simulink model "RobotControl1"  (R2015a)
settings: Solver=ode3  StartTime=0.0  StopTime=inf  FixedStep=1/7.5  RelTol=1e-3
undefined symbols (not defined in the file or in its folder): RGB24
libraries: slrtlib x12, xpcvideousblib x3, AAxpcseriallibold x3, xpcobsoletelib x2, rtvideolib x1, xpcutilitieslib x1
settings Model: SimulationMode=external  Creator=farbod  LastModifiedBy=sd0016
settings SolverCC: EnableConcurrentExecution=on
settings DataIOCC: SignalLoggingSaveFormat=ModelDataLogs
settings OptimizationCC: BlockReduction=off  OptimizeBlockIOStorage=off  BufferReuse=off  GlobalBufferReuse=off  ExpressionFolding=off  ExpressionDepthLimit=2147483647  LocalBlockOutputs=off
settings DebuggingCC: UnderspecifiedInitializationDetection=Classic  MergeDetectMultiDrivingBlocksExec=none  FcnCallInpInsideContextMsg=UseLocalSettings  StateNameClashWarn=warning
settings HardwareCC: ProdIntDivRoundTo=Zero  ProdEndianess=LittleEndian  ProdLongLongMode=on  ProdHWDeviceType=Generic->32-bit x86 compatible  TargetBitPerLong=64  TargetBitPerPointer=64  TargetIntDivRoundTo=Zero  TargetEndianess=LittleEndian  TargetWordSize=64  TargetHWDeviceType=Intel->x86-64
settings SFSimCC: SimParseCustomCode=off
settings RTWCC: SystemTargetFile=slrt.tlc  TemplateMakefile=slrt_default_tmf  Description=Simulink Real-Time  RTWVerbose=off  RTWCompilerOptimization=on
settings CodeAppCC: MaxIdLength=95
settings SimulinkRealTimeCC: GeneratePreprocessorConditionals=Disable all

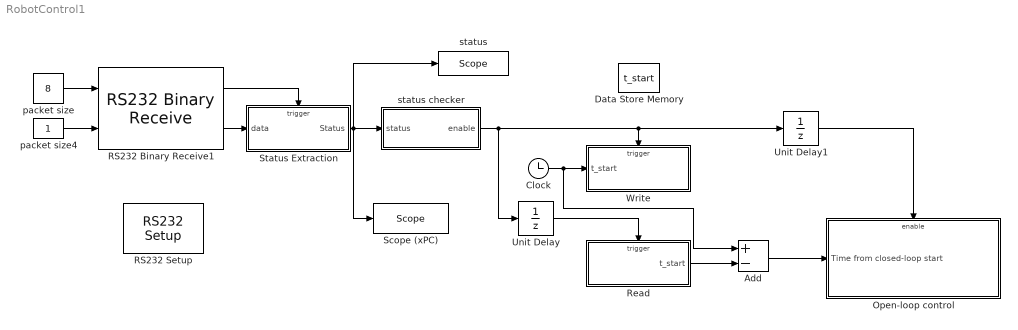
== system RobotControl1 ==
  Add : Sum  Inputs=+-
  Clock : Clock
  Data Store Memory : DataStoreMemory  DataStoreName=t_start  ReadBeforeWriteMsg=warning  WriteAfterWriteMsg=warning  WriteAfterReadMsg=warning
  Open-loop control : Subsystem
  RS232 Binary Receive1 : AAxpcseriallibold/Obsolete/Binary Mode/RS232 Binary Receive  port=COM1  width=8  samptime=-1
  "RS232 Setup " : AAxpcseriallibold/Obsolete/RS232 Setup   port=COM1  baud=115200  dbits=8  sbits=1  parity=None  prot=None  sbuf=2048  rbuf=2048  initstruct=[]  termstruct=[]
  Read : Subsystem  TreatAsAtomicUnit=on
  "Scope (xPC) " : slrtlib/Displays and Logging/Scope   scopeno=20  scopetype=Target  autostart=on  viewmode=Graphical rolling  formatstr='status=%3.3f'  grid=on  ylimits=[0,0]  nosamples=2000  noprepostsamples=0  interleave=1  triggermode=FreeRun  triggersignal=1  trigsignalfromport=off  triggerlevel=0.0  triggerslope=Either  triggerscope=1  triggersample=0  filename=data.dat  mode=Lazy  writesize=512  autorestart=off  dynamicfilemode=off  maxwritefilesize=512*1024^2
  Status Extraction : Subsystem  TreatAsAtomicUnit=on
  Unit Delay : UnitDelay  SampleTime=-1
  Unit Delay1 : UnitDelay  SampleTime=-1
  Write : Subsystem  TreatAsAtomicUnit=on
  packet size : Constant  Value=8
  packet size4 : Constant
  status : slrtlib/Displays and Logging/Scope   scopeno=6  scopetype=File  autostart=on  viewmode=Graphical rolling  formatstr='%15.6f'  grid=on  ylimits=[-10,50]  nosamples=3000  noprepostsamples=0  interleave=1  triggermode=FreeRun  triggersignal=1  trigsignalfromport=off  triggerlevel=0.0  triggerslope=Either  triggerscope=1  triggersample=0  filename=1sttus01.dat  mode=Commit  writesize=512  autorestart=on  dynamicfilemode=off  maxwritefilesize=512*1024^2
  status checker : MATLAB Function  TreatAsAtomicUnit=on
  wires:
  Unit Delay/1 -> Read/Trigger
  Clock/1 -> Write/1(t_start), Add/1
  Read/1(t_start) -> Add/2
  Status Extraction/1(Status) -> status/1, "Scope (xPC) "/1, status checker/1(status)
  status checker/1(enable) -> Write/Trigger, Unit Delay1/1, Unit Delay/1
  Unit Delay1/1 -> Open-loop control/Enable
  Add/1 -> Open-loop control/1(Time from closed-loop start)
  RS232 Binary Receive1/2 -> Status Extraction/1(data)
  RS232 Binary Receive1/1 -> Status Extraction/Trigger
  packet size4/1 -> RS232 Binary Receive1/2
  packet size/1 -> RS232 Binary Receive1/1

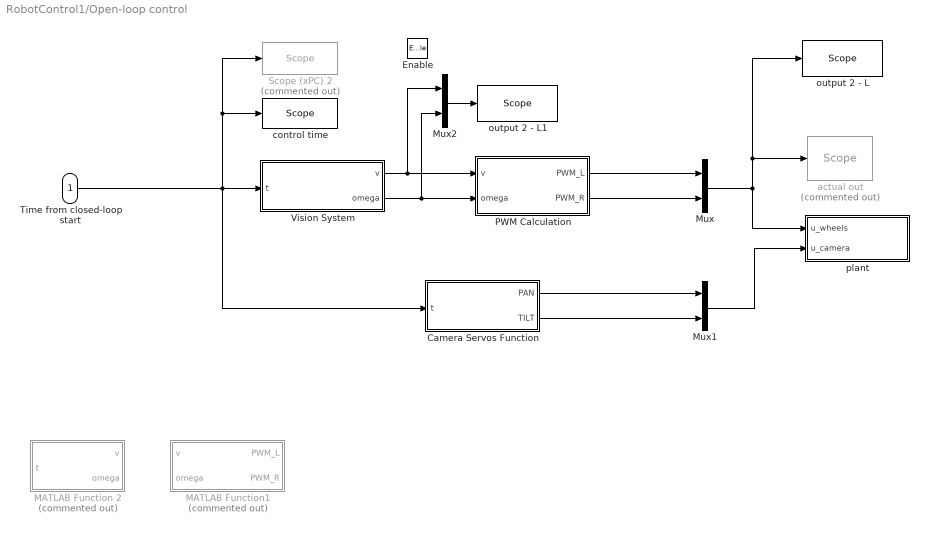
== system RobotControl1/Open-loop control ==
  Time from closed-loop start : Inport
  Enable : EnablePort  PropagateVarSize=During execution
  " MATLAB Function1" : MATLAB Function  Commented=on  TreatAsAtomicUnit=on
  Camera Servos Function : MATLAB Function  TreatAsAtomicUnit=on
  MATLAB Function 2 : MATLAB Function  Commented=on  TreatAsAtomicUnit=on
  Mux : Mux  Inputs=2
  Mux1 : Mux  Inputs=2
  Mux2 : Mux  Inputs=2
  PWM Calculation : MATLAB Function  TreatAsAtomicUnit=on
  Scope (xPC) 2 : slrtlib/Displays and Logging/Scope   Commented=on  scopeno=1  scopetype=File  autostart=on  viewmode=Graphical redraw  formatstr='%15.6f'  grid=on  ylimits=[0,0]  nosamples=3000  noprepostsamples=0  interleave=1  triggermode=FreeRun  triggersignal=1  trigsignalfromport=off  triggerlevel=0.0  triggerslope=Either  triggerscope=1  triggersample=0  filename=1ctime01.dat  mode=Commit  writesize=512  autorestart=off  dynamicfilemode=off  maxwritefilesize=512*1024^2
  Vision System : Subsystem
  actual out : slrtlib/Displays and Logging/Scope   Commented=on  scopeno=7  scopetype=File  autostart=on  viewmode=Graphical rolling  formatstr='%15.6f'  grid=on  ylimits=[-3,150]  nosamples=3000  noprepostsamples=0  interleave=1  triggermode=FreeRun  triggersignal=1  trigsignalfromport=off  triggerlevel=0.0  triggerslope=Either  triggerscope=1  triggersample=0  filename=1pwm01.dat  mode=Commit  writesize=512  autorestart=on  dynamicfilemode=off  maxwritefilesize=512*1024^2
  control time : slrtlib/Displays and Logging/Scope   scopeno=15  scopetype=Target  autostart=on  viewmode=Numerical  formatstr='t=%3.3f'  grid=on  ylimits=[0,0]  nosamples=3  noprepostsamples=0  interleave=1  triggermode=FreeRun  triggersignal=1  trigsignalfromport=off  triggerlevel=0.0  triggerslope=Either  triggerscope=1  triggersample=0  filename=data.dat  mode=Lazy  writesize=512  autorestart=off  dynamicfilemode=off  maxwritefilesize=512*1024^2
  output 2 - L : slrtlib/Displays and Logging/Scope   scopeno=11  scopetype=Target  autostart=on  viewmode=Numerical  formatstr='%15.6f'  grid=on  ylimits=[0,0]  nosamples=3  noprepostsamples=0  interleave=1  triggermode=FreeRun  triggersignal=1  trigsignalfromport=off  triggerlevel=0.0  triggerslope=Either  triggerscope=1  triggersample=0  filename=data.dat  mode=Lazy  writesize=512  autorestart=off  dynamicfilemode=off  maxwritefilesize=512*1024^2
  output 2 - L1 : slrtlib/Displays and Logging/Scope   scopeno=10  scopetype=Target  autostart=on  viewmode=Numerical  formatstr='%15.6f'  grid=on  ylimits=[0,0]  nosamples=3  noprepostsamples=0  interleave=1  triggermode=FreeRun  triggersignal=1  trigsignalfromport=off  triggerlevel=0.0  triggerslope=Either  triggerscope=1  triggersample=0  filename=data.dat  mode=Lazy  writesize=512  autorestart=off  dynamicfilemode=off  maxwritefilesize=512*1024^2
  plant : Subsystem
  wires:
  Mux/1 -> output 2 - L/1, actual out/1, plant/1(u_wheels)
  Camera Servos Function/1(PAN) -> Mux1/1
  Camera Servos Function/2(TILT) -> Mux1/2
  Mux1/1 -> plant/2(u_camera)
  PWM Calculation/1(PWM_L) -> Mux/1
  PWM Calculation/2(PWM_R) -> Mux/2
  Time from closed-loop start/1 -> Vision System/1(t), Scope (xPC) 2/1, control time/1, Camera Servos Function/1(t)
  Vision System/2(omega) -> Mux2/2, PWM Calculation/2(omega)
  Vision System/1(v) -> Mux2/1, PWM Calculation/1(v)
  Mux2/1 -> output 2 - L1/1

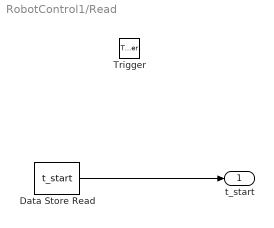
== system RobotControl1/Read ==
  Trigger : TriggerPort
  Data Store Read : DataStoreRead  DataStoreName=t_start
  t_start : Outport
  wires:
  Data Store Read/1 -> t_start/1

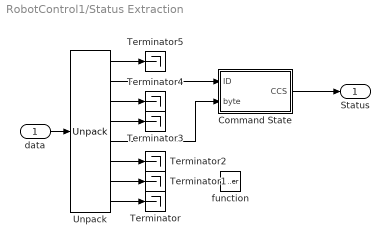
== system RobotControl1/Status Extraction ==
  data : Inport
  function : TriggerPort  TriggerType=function-call  OutputDataType=int8
  Command State : MATLAB Function  TreatAsAtomicUnit=on
  Terminator{,1..5} (6 alike) : Terminator
  Unpack : xpcobsoletelib/Utilities/Unpack   dimensions={1,1,1,1,1,1,1,1}  datatypes={'uint8','uint8','uint8','uint8','uint8','uint8','uint8','uint8'}  byteAlign=1
  Status : Outport
  wires:
  data/1 -> Unpack/1
  Command State/1(CCS) -> Status/1
  Unpack/5 -> Command State/2(byte)
  Unpack/2 -> Command State/1(ID)
  Unpack/8 -> Terminator/1
  Unpack/1 -> Terminator5/1
  Unpack/3 -> Terminator4/1
  Unpack/4 -> Terminator3/1
  Unpack/6 -> Terminator2/1
  Unpack/7 -> Terminator1/1

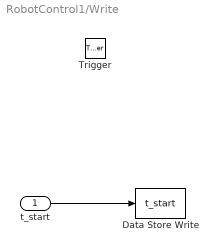
== system RobotControl1/Write ==
  t_start : Inport
  Trigger : TriggerPort
  Data Store Write : DataStoreWrite  DataStoreName=t_start
  wires:
  t_start/1 -> Data Store Write/1

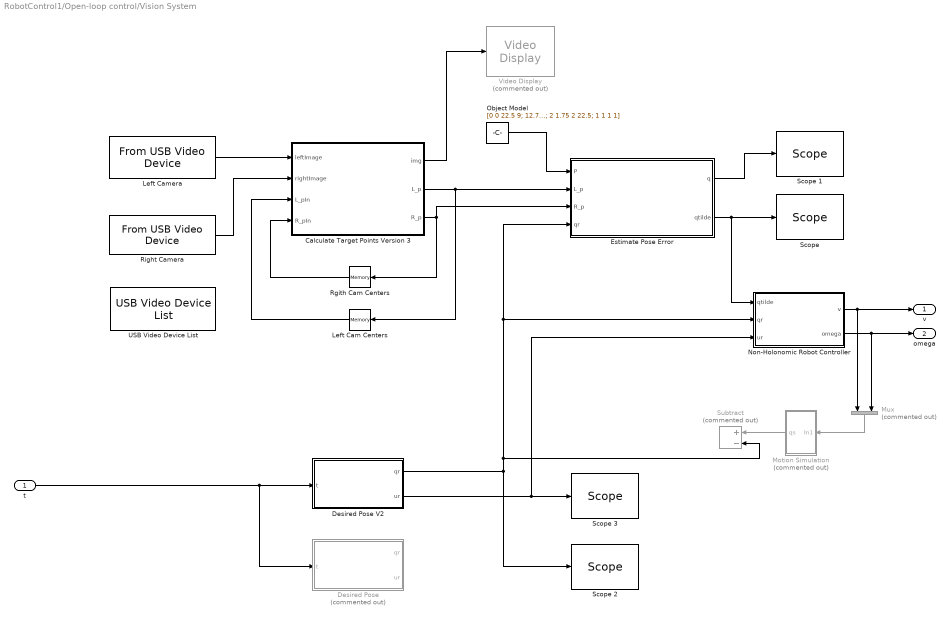
== system RobotControl1/Open-loop control/Vision System ==
  t : Inport
  Calculate Target Points Version 3 : MATLAB Function  TreatAsAtomicUnit=on
  Desired Pose : MATLAB Function  Commented=on  TreatAsAtomicUnit=on
  Desired Pose V2 : MATLAB Function  TreatAsAtomicUnit=on
  Estimate Pose Error : MATLAB Function  TreatAsAtomicUnit=on
  Left Cam Centers : Memory  X0=|  InheritSampleTime=on
      | [648.8644  845.2955  739.9159  733.5896;
      |   524.5901  515.6750  499.5366  358.6522]
  Left Camera : xpcvideousblib/From USB Video Device  sconf=<Select a configuration>  paddr=1.0  iwidth=1280  iheight=960  fint=1/7.5  ffmt=Uncompressed  cfmt=RGB24 (8:8:8)  isig=One multidimensional signal  trigger=off  status=off  updateBlock=1
  Motion Simulation : Subsystem  Commented=on
  Mux : Mux  Commented=on  Inputs=2
  Non-Holonomic Robot Controller : MATLAB Function  TreatAsAtomicUnit=on
  Object Model : Constant  Value=[0 0 22.5 9; 12.75 -12.75 0 0; 2 1.75 2 22.5; 1 1 1 1]
  Rgith Cam Centers : Memory  X0=|  InheritSampleTime=on
      | [560.7818  756.9749  660.6839  646.1424;
      |   602.0955  590.6171  575.2937  435.0033]
  Right Camera : xpcvideousblib/From USB Video Device  sconf=<Select a configuration>  paddr=1.3  iwidth=1280  iheight=960  fint=1/7.5  ffmt=Uncompressed  cfmt=RGB24 (8:8:8)  isig=One multidimensional signal  trigger=off  status=off  updateBlock=1
  "Scope " : slrtlib/Displays and Logging/Scope   scopeno=3  scopetype=Target  autostart=on  viewmode=Numerical  formatstr='%15.6f'  grid=on  ylimits=[0,0]  nosamples=3  noprepostsamples=0  interleave=1  triggermode=FreeRun  triggersignal=1  trigsignalfromport=off  triggerlevel=0.0  triggerslope=Either  triggerscope=1  triggersample=0  filename=data.dat  mode=Lazy  writesize=512  autorestart=off  dynamicfilemode=off  maxwritefilesize=512*1024^2
  Scope 1 : slrtlib/Displays and Logging/Scope   scopeno=1  scopetype=Target  autostart=on  viewmode=Numerical  formatstr='%15.6f'  grid=on  ylimits=[0,0]  nosamples=3  noprepostsamples=0  interleave=1  triggermode=FreeRun  triggersignal=1  trigsignalfromport=off  triggerlevel=0.0  triggerslope=Either  triggerscope=1  triggersample=0  filename=q.dat  mode=Lazy  writesize=512  autorestart=off  dynamicfilemode=off  maxwritefilesize=512*1024^2
  Scope 2 : slrtlib/Displays and Logging/Scope   scopeno=2  scopetype=Target  autostart=on  viewmode=Numerical  formatstr='%15.6f'  grid=on  ylimits=[0,0]  nosamples=3  noprepostsamples=0  interleave=1  triggermode=FreeRun  triggersignal=1  trigsignalfromport=off  triggerlevel=0.0  triggerslope=Either  triggerscope=1  triggersample=0  filename=data.dat  mode=Lazy  writesize=512  autorestart=off  dynamicfilemode=off  maxwritefilesize=512*1024^2
  Scope 3 : slrtlib/Displays and Logging/Scope   scopeno=9  scopetype=Target  autostart=on  viewmode=Numerical  formatstr='%15.6f'  grid=on  ylimits=[0,0]  nosamples=3  noprepostsamples=0  interleave=1  triggermode=FreeRun  triggersignal=1  trigsignalfromport=off  triggerlevel=0.0  triggerslope=Either  triggerscope=1  triggersample=0  filename=data.dat  mode=Lazy  writesize=512  autorestart=off  dynamicfilemode=off  maxwritefilesize=512*1024^2
  Subtract : Sum  Commented=on  Inputs=+-
  USB Video Device List : xpcvideousblib/USB Video Device List  usb_search=on  ShowInLibBrowser=0
  Video Display : rtvideolib/Video Display  Commented=on  imagesignal=Single multidimensional signal  colorspace=RGB  vindex=1
  v : Outport
  omega : Outport  Port=2
  wires:
  t/1 -> Desired Pose V2/1(t), Desired Pose/1(t)
  Non-Holonomic Robot Controller/1(v) -> v/1, Mux/1
  Non-Holonomic Robot Controller/2(omega) -> omega/1, Mux/2
  Object Model/1 -> Estimate Pose Error/1(P)
  Calculate Target Points Version 3/2(L_p) -> Left Cam Centers/1, Estimate Pose Error/2(L_p)
  Calculate Target Points Version 3/3(R_p) -> Rgith Cam Centers/1, Estimate Pose Error/3(R_p)
  Left Cam Centers/1 -> Calculate Target Points Version 3/3(L_pIn)
  Rgith Cam Centers/1 -> Calculate Target Points Version 3/4(R_pIn)
  Left Camera/1 -> Calculate Target Points Version 3/1(leftImage)
  Right Camera/1 -> Calculate Target Points Version 3/2(rightImage)
  Estimate Pose Error/2(qtilde) -> Non-Holonomic Robot Controller/1(qtilde), "Scope "/1
  Calculate Target Points Version 3/1(img) -> Video Display/1
  Estimate Pose Error/1(q) -> Scope 1/1
  Desired Pose V2/2(ur) -> Scope 3/1, Non-Holonomic Robot Controller/3(ur)
  Desired Pose V2/1(qr) -> Non-Holonomic Robot Controller/2(qr), Estimate Pose Error/4(qr), Subtract/2, Scope 2/1
  Mux/1 -> Motion Simulation/1(In1)
  Motion Simulation/1(qs) -> Subtract/1

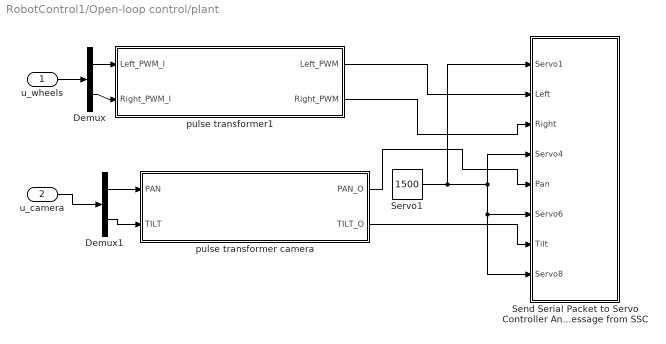
== system RobotControl1/Open-loop control/plant ==
  u_wheels : Inport
  u_camera : Inport  Port=2
  Demux : Demux  Outputs=2
  Demux1 : Demux  Outputs=2
  Send Serial Packet to Servo Controller And recieve status message from SSC : Subsystem  TreatAsAtomicUnit=on
  Servo1 : Constant  Value=1500  OutDataTypeStr=uint16
  pulse transformer camera : MATLAB Function  TreatAsAtomicUnit=on
  pulse transformer1 : MATLAB Function  TreatAsAtomicUnit=on
  wires:
  Servo1/1 -> Send Serial Packet to Servo Controller And recieve status message from SSC/6(Servo6), Send Serial Packet to Servo Controller And recieve status message from SSC/8(Servo8), Send Serial Packet to Servo Controller And recieve status message from SSC/4(Servo4), Send Serial Packet to Servo Controller And recieve status message from SSC/1(Servo1)
  u_wheels/1 -> Demux/1
  Demux/1 -> pulse transformer1/1(Left_PWM_I)
  Demux/2 -> pulse transformer1/2(Right_PWM_I)
  u_camera/1 -> Demux1/1
  pulse transformer1/1(Left_PWM) -> Send Serial Packet to Servo Controller And recieve status message from SSC/2(Left)
  pulse transformer1/2(Right_PWM) -> Send Serial Packet to Servo Controller And recieve status message from SSC/3(Right)
  Demux1/1 -> pulse transformer camera/1(PAN)
  Demux1/2 -> pulse transformer camera/2(TILT)
  pulse transformer camera/1(PAN_O) -> Send Serial Packet to Servo Controller And recieve status message from SSC/5(Pan)
  pulse transformer camera/2(TILT_O) -> Send Serial Packet to Servo Controller And recieve status message from SSC/7(Tilt)

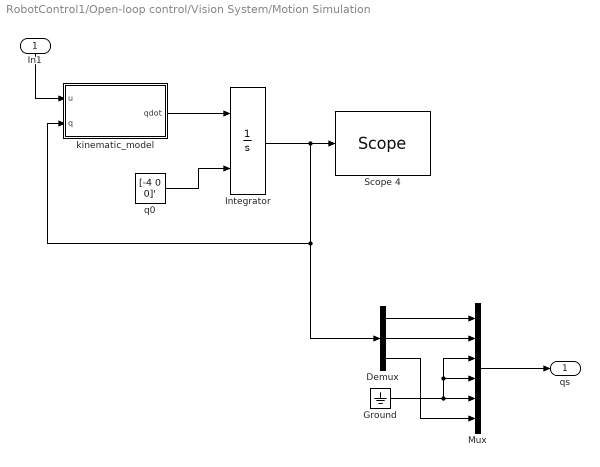
== system RobotControl1/Open-loop control/Vision System/Motion Simulation ==
  In1 : Inport
  Demux : Demux  Outputs=3
  Ground : Ground
  Integrator : Integrator  InitialConditionSource=external
  Mux : Mux  Inputs=6
  Scope 4 : slrtlib/Displays and Logging/Scope   scopeno=30  scopetype=File  autostart=on  viewmode=Graphical rolling  formatstr='%15.6f'  grid=on  ylimits=[0,0]  nosamples=250  noprepostsamples=0  interleave=1  triggermode=FreeRun  triggersignal=1  trigsignalfromport=off  triggerlevel=0.0  triggerslope=Either  triggerscope=1  triggersample=0  filename=data.dat  mode=Lazy  writesize=512  autorestart=off  dynamicfilemode=off  maxwritefilesize=512*1024^2
  kinematic_model : MATLAB Function  TreatAsAtomicUnit=on
  q0 : Constant  Value=[-4 0 0]'
  qs : Outport
  wires:
  kinematic_model/1(qdot) -> Integrator/1
  In1/1 -> kinematic_model/1(u)
  Integrator/1 -> Demux/1, kinematic_model/2(q), Scope 4/1
  q0/1 -> Integrator/2
  Mux/1 -> qs/1
  Demux/1 -> Mux/1
  Demux/2 -> Mux/2
  Demux/3 -> Mux/6
  Ground/1 -> Mux/5, Mux/3, Mux/4

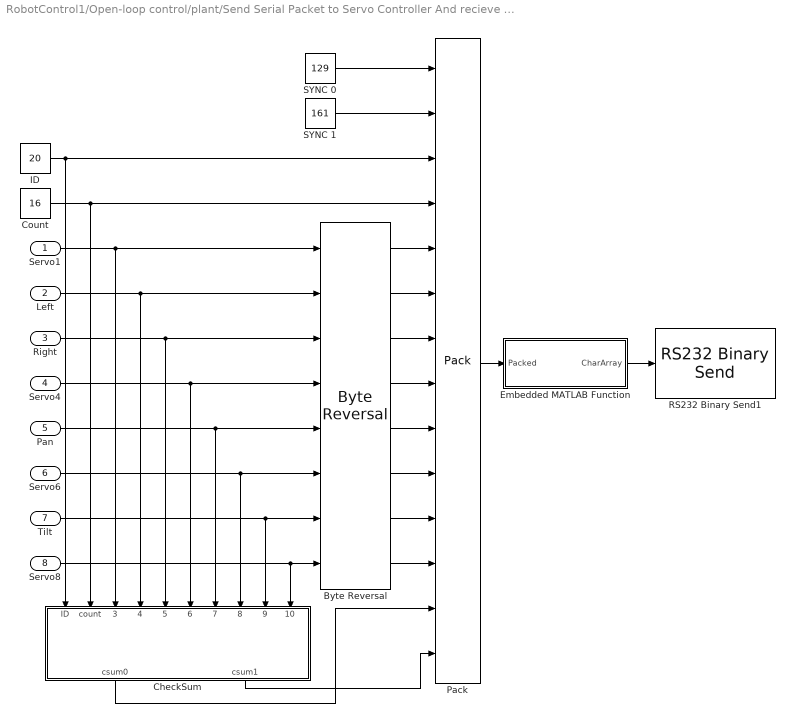
== system RobotControl1/Open-loop control/plant/Send Serial Packet to Servo Controller And recieve status message from SSC ==
  Servo1 : Inport  OutDataTypeStr=uint16
  Left : Inport  Port=2  OutDataTypeStr=uint16
  Right : Inport  Port=3  OutDataTypeStr=uint16
  Servo4 : Inport  Port=4  OutDataTypeStr=uint16
  Pan : Inport  Port=5  OutDataTypeStr=uint16
  Servo6 : Inport  Port=6  OutDataTypeStr=uint16
  Tilt : Inport  Port=7  OutDataTypeStr=uint16
  Servo8 : Inport  Port=8  OutDataTypeStr=uint16
  Byte Reversal : xpcutilitieslib/Byte Reversal   numInp=8
  CheckSum : MATLAB Function  TreatAsAtomicUnit=on
  Count : Constant  Value=16  OutDataTypeStr=uint8
  Embedded MATLAB Function : MATLAB Function  TreatAsAtomicUnit=on
  ID : Constant  Value=20  OutDataTypeStr=uint8
  Pack : xpcobsoletelib/Utilities/Pack   datatypes={'uint8','uint8','uint8','uint8','uint16','uint16','uint16','uint16','uint16','uint16','uint16','uint16','uint8','uint8'}  byteAlign=1
  RS232 Binary Send1 : AAxpcseriallibold/Obsolete/Binary Mode/RS232 Binary Send  port=COM1  width=22  samptime=-1
  SYNC 0 : Constant  Value=129  OutDataTypeStr=uint8
  SYNC 1 : Constant  Value=161  OutDataTypeStr=uint8
  wires:
  SYNC 0/1 -> Pack/1
  SYNC 1/1 -> Pack/2
  ID/1 -> Pack/3, CheckSum/1(ID)
  Count/1 -> Pack/4, CheckSum/2(count)
  Byte Reversal/2 -> Pack/6
  Byte Reversal/1 -> Pack/5
  Byte Reversal/3 -> Pack/7
  Byte Reversal/4 -> Pack/8
  Byte Reversal/5 -> Pack/9
  Byte Reversal/6 -> Pack/10
  Byte Reversal/7 -> Pack/11
  Byte Reversal/8 -> Pack/12
  CheckSum/2(csum1) -> Pack/14
  CheckSum/1(csum0) -> Pack/13
  Servo8/1 -> Byte Reversal/8, CheckSum/10(servo8)
  Tilt/1 -> Byte Reversal/7, CheckSum/9(servo7)
  Servo6/1 -> Byte Reversal/6, CheckSum/8(servo6)
  Pan/1 -> Byte Reversal/5, CheckSum/7(servo5)
  Servo4/1 -> Byte Reversal/4, CheckSum/6(servo4)
  Right/1 -> Byte Reversal/3, CheckSum/5(servo3)
  Left/1 -> Byte Reversal/2, CheckSum/4(servo2)
  Servo1/1 -> Byte Reversal/1, CheckSum/3(servo1)
  Pack/1 -> Embedded MATLAB Function/1(Packed)
  Embedded MATLAB Function/1(CharArray) -> RS232 Binary Send1/1

== matlab function RobotControl1/Open-loop control/MATLAB Function 2 ==
  data: t input; v output; omega output
function [v,omega] = fcn(t)
%#codegen

tau = 10;

v0 = 0.9;
omega0 = 0.5;

tshift = 1;

v = v0*sin(2*pi*t/tau);
omega = omega0*sin(2*pi*(t-tshift)/tau);

== matlab function RobotControl1/Open-loop control/Vision System/Non-Holonomic Robot Controller ==
  data: v output; qtilde input; qr input; ur input; omega output
function [v, omega] = controller(qtilde,qr,ur)
% the controller
% u = [v omega]^T
% qtilde: posture error
% qr    : reference (desired) posture

%%----------Input Parametleri Duzenleniyor---------------------------------

u = zeros(2,1);

% for now
vr     = ur(1,1);
omegar = ur(2,1);

% According to the vision system: qtilde = q - qr, so
q = qtilde + qr;

xr     = qr(1,1);
yr     = qr(2,1);
thetar = qr(6,1);

x     = q(1,1);
y     = q(2,1);
theta = q(6,1);

s = sin(theta);
c = cos(theta);

%% -------------------------Error Hesaplaniyor----------------------------
% Burada temelde 3 tane olan hata parametreleri 4 e cikariliyor. 
% theta parametresi es ve ec olarak iki ayri hata parametresine cevriliyor

% Eq.(4), third element!
etheta = thetar-theta;

% Local errors from Eq.(10)
ex = c*(xr - x) + s*(yr - y);
ey = -s*(xr - x) + c*(yr - y);

es = sin(thetar-theta);
ecos = cos(thetar-theta);

ec = ecos -1;

%--------------------------------------------------------------------------
%% - u ya ulasabilmek icin ihtiyacimiz olanlar
% vb,omegab,vr,omegar: ilk ikisi hesaplaniyor son ikisi ur'den geliyor.
% k,kx,ks,a,n paper temel alinarak secilmis secilmis

% according to the paper
k = 1; % k > 0
kx = 1; % kx(t) > 0
ks = 1; % ks(t) > 0
a = 3; % a > 2
n = 0; % n = -2, -1, 0, 1 or 2

% Eq.(18)
vb = kx*ex;
omegab = k*vr*ey*(1+ec/a)^2+ks*es*((1+ec/a)^2)^n;

v = (vr*cos(etheta)+vb); 
omega = omegar+omegab; % Eq.(6)

%buradaki u degeri controllerdan cikan ve sisteme giris olarak verilen u

== matlab function RobotControl1/Open-loop control/plant/Send Serial Packet to Servo Controller And recieve status message from SSC/CheckSum ==
  data: ID input; csum0 output; count input; servo1 input; servo2 input; csum1 output; servo3 input; servo4 input; servo5 input; servo6 input; servo7 input; servo8 input
function [csum0,csum1]= fcn(ID,count,servo1,servo2,servo3,servo4,servo5,servo6,servo7,servo8)
% The purpose of this function is to calculate the fletcher checksum values
% as defined in internet RFC 1145
% See page 11 of the Microbotics Servo Switch/Controller Users Manual for 
% more information

% break into bytes
servo1a=uint8(bitshift(servo1,-8)); servo1b=uint8(servo1-uint16(servo1a)*256);
servo2a=uint8(bitshift(servo2,-8)); servo2b=uint8(servo2-uint16(servo2a)*256);
servo3a=uint8(bitshift(servo3,-8)); servo3b=uint8(servo3-uint16(servo3a)*256);
servo4a=uint8(bitshift(servo4,-8)); servo4b=uint8(servo4-uint16(servo4a)*256);
servo5a=uint8(bitshift(servo5,-8)); servo5b=uint8(servo5-uint16(servo5a)*256);
servo6a=uint8(bitshift(servo6,-8)); servo6b=uint8(servo6-uint16(servo6a)*256);
servo7a=uint8(bitshift(servo7,-8)); servo7b=uint8(servo7-uint16(servo7a)*256);
servo8a=uint8(bitshift(servo8,-8)); servo8b=uint8(servo8-uint16(servo8a)*256);
byte=[ID, count, servo1a, servo1b, servo2a, servo2b, servo3a, servo3b, servo4a, servo4b, servo5a, servo5b, servo6a, servo6b, servo7a, servo7b, servo8a, servo8b];

cksum0=uint16(0);cksum1=uint16(0); % initialize to zero
for i=1:(count+2)
    cksum0=mod((cksum0+uint16(byte(i))),256);
    cksum1=mod((cksum1+cksum0),256);
end

csum0=uint8(cksum0); csum1=uint8(cksum1);

== matlab function RobotControl1/Open-loop control/ MATLAB Function1 ==
  data: v input; PWM_L output; omega input; PWM_R output
function [PWM_L,PWM_R] = fcn(v,omega)
%#codegen
v = -v;
omega = -omega;

T = 0.422;

vL = v -(T/2)*omega;
vR = v +(T/2)*omega;

vVec = [vL;vR];

aL = 3.8863614532;
bL = -0.0026808274;

aR = 3.2707294485;
bR = -0.0022447804;

A = [aL;aR];
B = [[bL,0];[0,bR]];

PWM = (B)\(vVec-A);

PWM_L = 1350;%PWM(1);
PWM_R = 1350;%PWM(2);

== matlab function RobotControl1/Open-loop control/Vision System/Desired Pose ==
  data: t input; qr output; ur output
function [qr,ur] = desired(t)
%#codegen

xr = -2.475;%vx*t - 30;
yr = 0; %A*sin(2*pi*xr/xL) + 2;
zr = 0.25;
phir = 0;
thetar = 0;

% desired x and y derivatives
xrdot = 0; %vx;
yrdot = 0; %A*(2*pi/xL)*cos(2*pi*xr/xL);

% desired theta
psir = atan2(yrdot,xrdot);

% desired second derivatives
xrddot = 0;
yrddot = 0;%-A*(2*pi/xL)^2*sin(2*pi*xr/xL);

% desired theta derivative
thetardot = 0;%(yrddot - xrddot*tan(thetar))/(xrdot*(1+tan(thetar)^2));

vr     = sqrt(xrdot^2+yrdot^2);
omegar = thetardot;

qr = [xr;yr;zr;phir;thetar;psir];
ur = [vr;omegar];

== matlab function RobotControl1/Open-loop control/Vision System/Calculate Target Points Version 3 ==
  data: img output; leftImage input; L_p output; rightImage input; L_pIn input; R_pIn input; R_p output
function [img,L_p, R_p] = getCenterV3(leftImage, rightImage, L_pIn, R_pIn)
    %#codegen 
    ps = 0; %Pad Size
%     leftImage = padarray(leftImage,[ps ps],'both');
%     rightImage = padarray(rightImage,[ps ps],'both');
    
    lwc = round(L_pIn) + ps; %Center of the left windows
    rwc = round(R_pIn) + ps; %Center of the right windows
    
    L_p = zeros(2,4);
    R_p = zeros(2,4);
    
    winRng = -40:40;
    n = length(winRng);
    
    img = uint8(zeros(2*n,4*n));
    
    for i=1:4
        lwx = winRng + lwc(1,i);
        lwy = winRng + lwc(2,i);
        
        rwx = winRng + rwc(1,i);
        rwy = winRng + rwc(2,i);
        
        pWinL = leftImage(lwy,lwx,:);
        pWinR = rightImage(rwy,rwx,:);
                
        pWinL = imcomplement(pWinL);        
        pWinR = imcomplement(pWinR);        
            
        pGrayL = 0.2989 * pWinL(:,:,1) + 0.5870 * pWinL(:,:,2) + 0.1140 * pWinL(:,:,3);
        pGrayR = 0.2989 * pWinR(:,:,1) + 0.5870 * pWinR(:,:,2) + 0.1140 * pWinR(:,:,3);
    
        pWinLF = pWinL(:,:,3) - pGrayL;       % imsubtract(rgb1(:,:,3),gray)
        pWinRF = pWinR(:,:,3) - pGrayR;       % imsubtract(rgb1(:,:,3),gray) 
        
        rng = (1:n) + (i-1)*n;
        img(1:n,rng) = pGrayL;
        img(n+1:end,rng) = pGrayR;
        
        hautoth = vision.Autothresholder;
        pBWL = step(hautoth,pWinLF);
        pBWR = step(hautoth,pWinRF);
        
        %finds yellow regions in image using BlobAnalysis.
        hblob = vision.BlobAnalysis;

        [aL,cL,~] = step(hblob, pBWL); % get [x y] is a centroid of region
        [aR,cR,~] = step(hblob, pBWR); % get [x y] is a centroid of region
        
        [~, indL] = sort(aL,'descend');
        [~, indR] = sort(aR,'descend');
        
        if(size(cL,1) ~= 0) && (size(cR,1) ~= 0)
            L_p(:,i) = cL(indL(1),:)' + [lwx(1);lwy(1)] - [ps;ps];
            R_p(:,i) = cR(indR(1),:)' + [rwx(1);rwy(1)] - [ps;ps];
        else
            L_p(:,i) = L_pIn(:,i);
            R_p(:,i) = R_pIn(:,i);
        end 
    end
end

== matlab function RobotControl1/Open-loop control/Vision System/Estimate Pose Error ==
  data: q output; P input; L_p input; R_p input; qr input; qtilde output
function [q, qtilde] = mirage(P,L_p,R_p,qr)
%#codegen

%Desired Robot Pose for current step qr()
robotPoseDes.x = qr(1);
robotPoseDes.y = qr(2);
robotPoseDes.z = qr(3);
robotPoseDes.phi = qr(4);
robotPoseDes.theta = qr(5);
robotPoseDes.psi = qr(6);

%Transform target points from I space into Desired Robot Space
world2robotDes = inv(EulerTrans(robotPoseDes));
S_PDes = world2robotDes*P;

%Calculate the error parameters for current step
errParams = visioMotor(L_p,R_p,S_PDes);

poseErrorMat = eye(4,4);
poseErrorMat(1:3,:) = reshape(errParams,3,4);

world2robot = poseErrorMat*world2robotDes;

robotPoseEst = calculatePose(world2robot);

q = [-robotPoseEst.x/100 -robotPoseEst.y/100 -robotPoseEst.z/100 -robotPoseEst.phi   -robotPoseEst.theta -robotPoseEst.psi]';

qtilde = [ -robotPoseEst.x/100  - robotPoseDes.x;
           -robotPoseEst.y/100  - robotPoseDes.y;
           -robotPoseEst.z/100  - robotPoseDes.z;
           -robotPoseEst.phi  - robotPoseDes.phi;
           -robotPoseEst.theta  - robotPoseDes.theta;
           -robotPoseEst.psi  - robotPoseDes.psi;];
       
end

== matlab function RobotControl1/Open-loop control/Vision System/Desired Pose V2 ==
  data: t input; qr output; ur output
function [qr, ur] = desired(t)
%#codegen

    x0 = 1.87;
    xc = 0.95;
    T = 12;
    
%     if(t > 12)
%         t = 12;
%     end

    t = 0;
    
    %Position/Time
    xr = -(x0+xc)/2 - (x0-xc)/2*cos(2*pi*t/T);
    yr = 0;
    zr = 0.25;
    phir = 0;
    thetar = 0;
     
    xrdot = (61*pi*sin((pi*t)/6))/240;
    yrdot = 0;
    
    psir = atan2(yrdot,xrdot);
    
    % desired second derivatives
    xrddot = (61*pi^2*cos((pi*t)/6))/1440;
    yrddot = 0;
    
    if(xrdot == 0)
        xrdot = 0.01;
    end
    
    % desired theta derivative
    thetardot = (yrddot - xrddot*tan(thetar))/(xrdot*(1+tan(thetar)^2));

    vr     = sqrt(xrdot^2+yrdot^2);
    omegar = thetardot;
    
    qr = [xr yr zr phir thetar psir]';
    ur = [vr omegar]';
end

== matlab function RobotControl1/Open-loop control/Vision System/Motion Simulation/kinematic_model ==
  data: u input; q input; qdot output
function qdot = kinematic(u,q)
% Kinematic Model

% q = [x y theta]^T
% qdot = [xdot ydot thetadot]^T
% u = [v omega]^T

qdot = zeros(3,1);

theta = q(3);
qdot = [cos(theta),0;sin(theta),0;0,1]*u; % Eq.(2)

== matlab function RobotControl1/Open-loop control/PWM Calculation ==
  data: v input; PWM_L output; omega input; PWM_R output
function [PWM_L, PWM_R] = PWM(v, omega)
%#codegen

T = 0.422;

vL = v -(T/2)*omega;
vR = v +(T/2)*omega;

%----------------------------------
%Calculations for left wheel motor
if(vL < -1.64)
    PWM_L = 1000;
    
elseif(vL < 0)
    %function for the negative area
    PWM_L = 97.06*vL^3 + 332.9*vL^2 + 525.5*vL + 1395;
    
elseif(vL < 1.73)
    %function for the positive area
    PWM_L = 33.26*vL^3 + -144.5*vL^2 + 384.7*vL + 1593;
    
else
    PWM_L = 2000;
    
end

%----------------------------------
%Calculations for right wheel motor
if(vR < -1.66)
    PWM_R = 1000;
    
elseif(vR < 0)
    %function for negative area
    PWM_R = 74.33*vR^3 + 276.6*vR^2 + 492.8*vR + 1397;
    
elseif(vR < 1.72)
    %function for positve area
    PWM_R = 39.94*vR^3 + -175.9*vR^2 + 419.6*vR + 1594;
    
else
    PWM_R = 2000;
    
end

== matlab function RobotControl1/Open-loop control/Camera Servos Function ==
  data: t input; PAN output; TILT output
 function [PAN,TILT] = fcn(t)
%Insert Function for camera servo manipulation here
%By default, this function holds camera servos at their center position (1500 ms)
PAN = 1525;
TILT = 1400;

== matlab function RobotControl1/Open-loop control/plant/pulse transformer camera ==
  data: PAN input; TILT input; PAN_O output; TILT_O output
function [PAN_O, TILT_O]  = fcn(PAN,TILT)

PAN_O  = uint16(PAN);
TILT_O = uint16(TILT);

== matlab function RobotControl1/Open-loop control/plant/pulse transformer1 ==
  data: Left_PWM_I input; Right_PWM_I input; Left_PWM output; Right_PWM output
function [Left_PWM, Right_PWM]  = fcn(Left_PWM_I,Right_PWM_I)
% This block supports an embeddable subset of the MATLAB language.
% Converts output angle and speed value into a pulse width
% The input angle is between +pi/4 and -pi/4  (from limits)
% The speed is between 140 and 0 rps(Hz)

% angle=uint16(angI*16.25*180/pi + 1505.5);
% pw=-0.0002*speedI^3 +0.03*speedI^2 -2.66*speedI +1528;
% throtle = uint16(pw);
% 
Left_PWM  = uint16(Left_PWM_I);
Right_PWM = uint16(Right_PWM_I);

== matlab function RobotControl1/Status Extraction/Command State ==
  data: ID input; CCS output; byte input
function CCS = fcn(ID, byte)
% This block supports an embeddable subset of the MATLAB language.
% See the help menu for details. 
% outputs the command channel state (CCS) given status output

% first check that have proper status message
% ID = 10 for SSC status info
if ID==10
    if byte==2
        out=1;
    elseif byte==4;
        out=2;
    elseif byte==6
        out=3;
    else
        out=0;
    end
else
    out=4;
end
CCS = out;

== matlab function RobotControl1/status checker ==
  data: status input; enable output
function enable = fcn(status)
% This block supports an embeddable subset of the MATLAB language.
% See the help menu for details. 
if status==1  
    en = 1;
else
    en = -1;
end
enable=en;

== matlab function RobotControl1/Open-loop control/plant/Send Serial Packet to Servo Controller And recieve status message from SSC/Embedded MATLAB Function ==
  data: Packed input; CharArray output
function CharArray = fcn(Packed)
%
CharArray = zeros(22,1,'uint8');
CharArray = Packed;
